simulink model "Copy_of_Admittance"  (R2023b)
settings: Solver=VariableStepAuto  StartTime=0.0  StopTime=10.0  RelTol=1e-3
InitFcn:
  | J=1e-6
  | B = 1e-6
values from neighbouring files (symbols this model uses):
  D = [0]    [motor_model_state_space.m]
  K = 1.10e-4    (= 0.00011)    [Admittance_code.m]    (also in motor_model_state_space.m = 100)
  Ke = 0.011    [Admittance_code.m]    (also in motor_model_state_space.m)
  Kt = 0.011    [Admittance_code.m]    (also in motor_model_state_space.m)
  L = 0.58E-3    (= 0.00058)    [Admittance_code.m]    (also in motor_model_state_space.m)
  M_inv = 1/J    (= 617283.950617)    [Admittance_code.m]    (also in motor_model_state_space.m = 1000000)
  R = 1.17    [Admittance_code.m]    (also in motor_model_state_space.m)
settings Model: Creator=sayeholoumi  LastModifiedBy=sayeholoumi

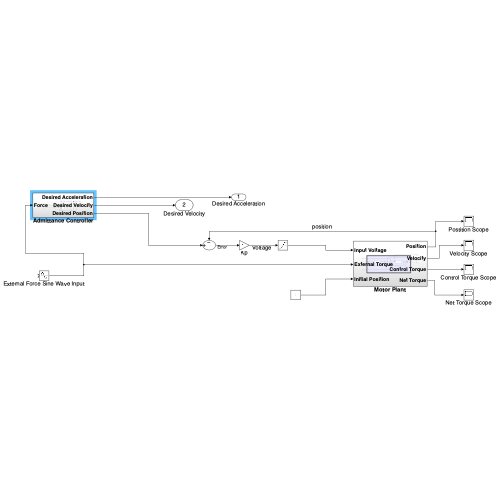
[thumbnail: Simulink's stored preview of the top-level diagram]
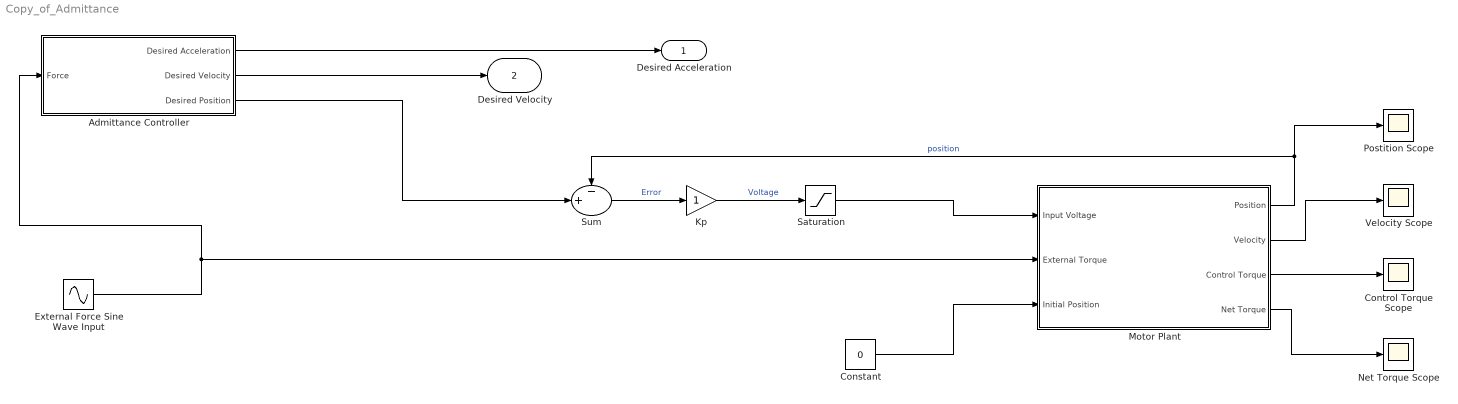
== system Copy_of_Admittance ==
  Admittance Controller : Subsystem
  Constant : Constant  Value=0
  Control Torque Scope : Scope
  External Force Sine Wave Input : Sin  TimeSource=Use external signal  SampleTime=0
  Kp : Gain
  Motor Plant : Subsystem
  Net Torque Scope : Scope
  Postition Scope : Scope
  Saturation : Saturate  UpperLimit=12  LowerLimit=-12
  Sum : Sum  Inputs=-+|
  Velocity Scope : Scope
  Desired Acceleration : Outport
  Desired Velocity : Outport  Port=2
  wires:
  Admittance Controller/1(Desired Acceleration) -> Desired Acceleration/1
  Admittance Controller/3(Desired Position) -> Sum/2
  Admittance Controller/2(Desired Velocity) -> Desired Velocity/1
  Constant/1 -> Motor Plant/3(Initial Position)
  External Force Sine Wave Input/1 -> Admittance Controller/1(Force), Motor Plant/2(External Torque)
  Motor Plant/1(Position) -> Postition Scope/1, Sum/1  "position"
  Kp/1 -> Saturation/1  "Voltage"
  Motor Plant/4(Net Torque) -> Net Torque Scope/1
  Motor Plant/3(Control Torque) -> Control Torque Scope/1
  Saturation/1 -> Motor Plant/1(Input Voltage)
  Motor Plant/2(Velocity) -> Velocity Scope/1
  Sum/1 -> Kp/1  "Error"

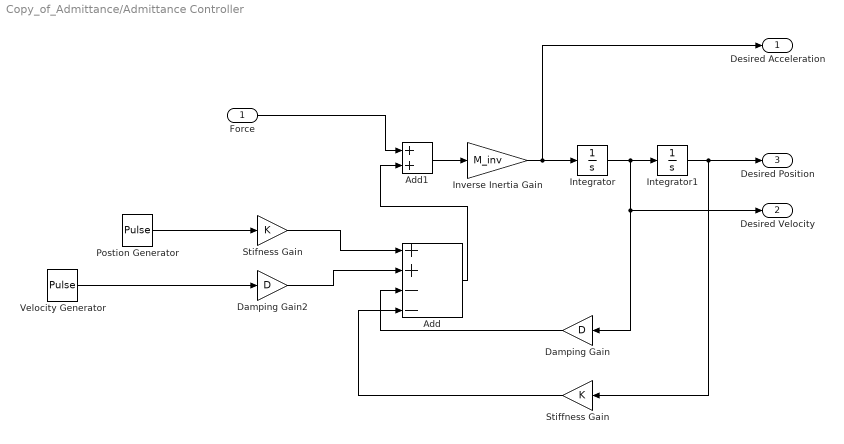
== system Copy_of_Admittance/Admittance Controller ==
  Force : Inport
  Add : Sum  Inputs=++--
  Add1 : Sum
  Damping Gain : Gain  Gain=D
  Damping Gain2 : Gain  Gain=D
  Integrator : Integrator
  Integrator1 : Integrator
  Inverse Inertia Gain : Gain  Gain=M_inv
  Postion Generator : DiscretePulseGenerator  PulseType=Time based  Period=10  PulseWidth=5
  "Stiffness Gain " : Gain  Gain=K
  Stifness Gain : Gain  Gain=K
  Velocity Generator : DiscretePulseGenerator  PulseType=Time based  Period=10  PulseWidth=5
  Desired Acceleration : Outport
  Desired Velocity : Outport  Port=2
  Desired Position : Outport  Port=3
  wires:
  Postion Generator/1 -> Stifness Gain/1
  Damping Gain2/1 -> Add/2
  Add/1 -> Add1/2
  Add1/1 -> Inverse Inertia Gain/1
  Damping Gain/1 -> Add/3
  Inverse Inertia Gain/1 -> Desired Acceleration/1, Integrator/1
  "Stiffness Gain "/1 -> Add/4
  Integrator1/1 -> Desired Position/1, "Stiffness Gain "/1
  Stifness Gain/1 -> Add/1
  Force/1 -> Add1/1
  Integrator/1 -> Desired Velocity/1, Damping Gain/1, Integrator1/1
  Velocity Generator/1 -> Damping Gain2/1

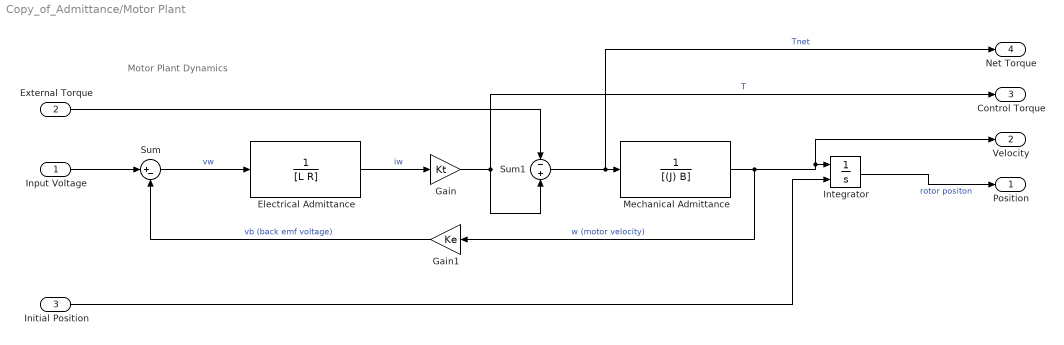
== system Copy_of_Admittance/Motor Plant ==
  note: Motor Plant Dynamics
  Input Voltage : Inport
  External Torque : Inport  Port=2
  Initial Position : Inport  Port=3
  Electrical Admittance : TransferFcn  Denominator=[L R]
  Gain : Gain  Gain=Kt
  Gain1 : Gain  Gain=Ke
  Integrator : Integrator  InitialConditionSource=external
  Mechanical Admittance : TransferFcn  Denominator=[(J) B]
  Sum : Sum  Inputs=|+-
  Sum1 : Sum  Inputs=-+
  Position : Outport
  Velocity : Outport  Port=2
  Control Torque : Outport  Port=3
  Net Torque : Outport  Port=4
  wires:
  Input Voltage/1 -> Sum/1
  Mechanical Admittance/1 -> Velocity/1, Integrator/1, Gain1/1  "w (motor velocity)"
  Gain1/1 -> Sum/2  "vb (back emf voltage)"
  Integrator/1 -> Position/1  "rotor positon"
  Gain/1 -> Control Torque/1, Sum1/2  "T"
  Electrical Admittance/1 -> Gain/1  "iw"
  Sum/1 -> Electrical Admittance/1  "vw"
  Sum1/1 -> Net Torque/1, Mechanical Admittance/1  "Tnet"
  External Torque/1 -> Sum1/1
  Initial Position/1 -> Integrator/2
